simulink subsystem "MPC3_opti"  (R2023b)
settings: Solver=VariableStepAuto  StartTime=0.0  StopTime=10.0  RelTol=1e-3
undefined symbols (not defined in the file): param_MPC3, param_robot, param_traj_data, param_weight_init
settings Model: Creator=emu  LastModifiedBy=emu

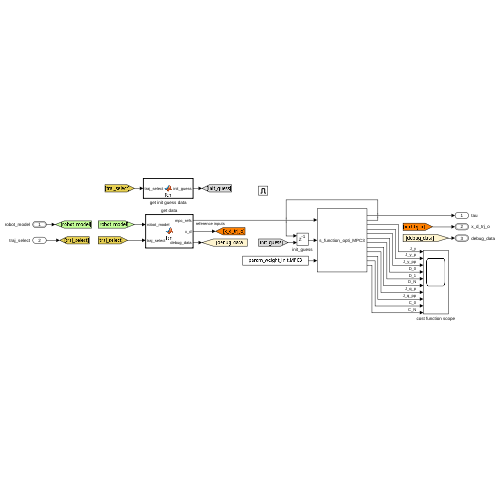
[thumbnail: Simulink's stored preview of the top-level diagram]
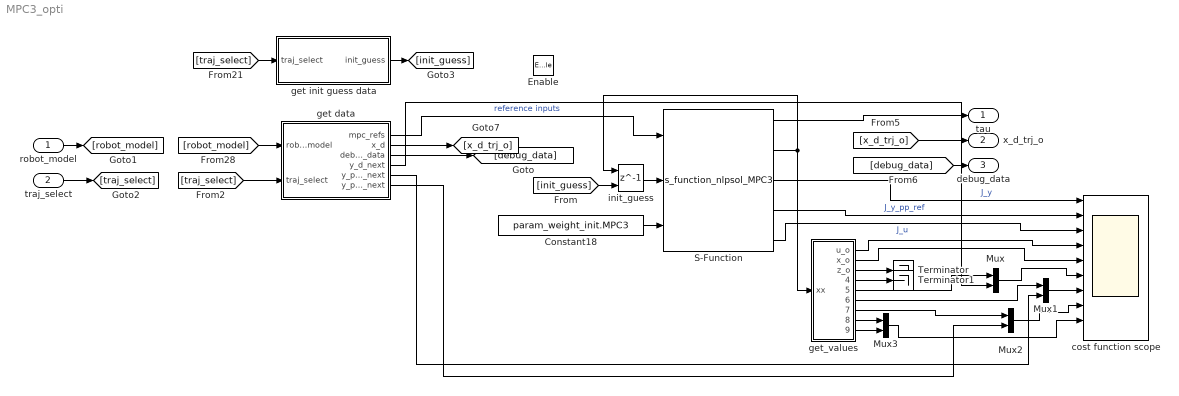
== system MPC3_opti ==
  robot_model : Inport  OutDataTypeStr=Bus: robot_model
  traj_select : Inport  Port=2
  Enable : EnablePort
  Constant18 : Constant  Value=param_weight_init.MPC3  VectorParams1D=off
  Mux{,1..3} (4 alike) : Mux  Inputs=2
  S-Function : S-Function  FunctionName=s_function_nlpsol_MPC3  Parameters='s_functions/MPC3.casadi', 'MPC3'  SFunctionModules='MPC3'  SFunctionDeploymentMode=off  EnableBusSupport=off
  Terminator : Terminator
  Terminator1 : Terminator
  cost function scope : Scope  NumInputPorts=10
  get data : MATLAB Function  TreatAsAtomicUnit=on
  get init guess data : MATLAB Function  TreatAsAtomicUnit=on
  get_values : MATLAB Function  TreatAsAtomicUnit=on
  init_guess : Delay  DelayLength=1  InitialConditionSource=Input port  InitialCondition=1
      settings: InputPortMap=u0,p4
  tau : Outport
  x_d_trj_o : Outport  Port=2  OutDataTypeStr=Bus: x_d
  debug_data : Outport  Port=3  OutDataTypeStr=Bus: debug_data_bus
  wires:
  get init guess data/1(init_guess) -> [init_guess]
  S-Function/2 -> init_guess/1, get_values/1(xx)
  [debug_data] -> debug_data/1
  get data/3(debug_data) -> [debug_data]
  get data/1(mpc_refs) -> S-Function/1  "reference inputs"
  S-Function/3 -> cost function scope/1  "J_y"
  [robot_model] -> get data/1(robot_model)
  S-Function/4 -> cost function scope/2  "J_y_pp_ref"
  [traj_select] -> get data/2(traj_select)
  [init_guess] -> init_guess/2
  Constant18/1 -> S-Function/3
  init_guess/1 -> S-Function/2
  [traj_select] -> get init guess data/1(traj_select)
  robot_model/1 -> [robot_model]
  [x_d_trj_o] -> x_d_trj_o/1
  get data/2(x_d) -> [x_d_trj_o]
  S-Function/1 -> tau/1
  traj_select/1 -> [traj_select]
  get_values/1(u_o) -> cost function scope/4
  get_values/2(x_o) -> cost function scope/5
  get_values/6(y_p_ref_next) -> Mux1/1
  get_values/7(y_pp_ref_next) -> Mux2/1
  get data/4(y_d_next) -> Mux/2
  get data/5(y_p_d_next) -> Mux1/2
  get data/6(y_pp_d_next) -> Mux2/2
  get_values/5(y_ref_next) -> Mux/1
  Mux1/1 -> cost function scope/7
  Mux2/1 -> cost function scope/8
  get_values/3(z_o) -> Terminator/1
  get_values/4(alpha_o) -> Terminator1/1
  Mux3/1 -> cost function scope/9
  get_values/8(y_N) -> Mux3/1
  get_values/9(y_ref_N) -> Mux3/2
  S-Function/5 -> cost function scope/3  "J_u"
  Mux/1 -> cost function scope/6

== matlab function MPC3_opti/get data ==
  settings: updateMethod=DISCRETE  sampleTime=param_global.Ta
  data: mpc_refs output; robot_model input Bus: robot_model; param_MPC3 parameter; x_d output Bus: x_d; debug_data output Bus: debug_data_bus; param_traj_data parameter; traj_select input; y_d_next output; y_p_d_next output; y_pp_d_next output
function [mpc_refs, x_d, debug_data, y_d_next, y_p_d_next, y_pp_d_next] = fcn(robot_model, param_MPC3, param_traj_data, traj_select)
persistent cnt;

if(isempty(cnt))
    cnt = 1;
end

param_MPC = param_MPC3;
N         = param_MPC.N;
N_step    = param_MPC.N_step;

% Parameters
q    = robot_model.q;      % generalized coordinates
q_p  = robot_model.q_p;  % time derivative of generalized coordinates
q_pp = robot_model.q_pp;
H    = robot_model.H;
J    = robot_model.J;
J_p  = robot_model.J_p;

% Current Pose of Endeffector
p = H(1:2,4);
p_p = J(1:2,1:2)*q_p;
p_pp = J(1:2,1:2)*q_pp + J_p(1:2,1:2)*q_p;

R = H(1:3,1:3);

% desired Orientation as Rotationmatrix
q_e = rotation2quaternion(R);

% Error of Position (translation) and first time derivative
q_err = quat_mult(q_e, quat_inv(param_traj_data.q_d(1:4, cnt, traj_select)));

x_k = [q;q_p];

% Assemble vector of recieved output measurements
p_d_traj    = param_traj_data.p_d(   1:3, cnt : N_step : cnt + (N)*N_step, traj_select);
p_d_p_traj  = param_traj_data.p_d_p( 1:3, cnt : N_step : cnt + (N)*N_step, traj_select);
p_d_pp_traj = param_traj_data.p_d_pp(1:3, cnt : N_step : cnt + (N)*N_step, traj_select);

y_ref    = p_d_traj(   1:2, 1 + (0:N) ); %       y1,   y2,   ... yN
y_ref_p  = p_d_p_traj( 1:2, 1 + (0:N) ); %       y1p,  y2p,  ... yNp
y_ref_pp = p_d_pp_traj(1:2, 1 + (0:N) ); % y0pp, y1pp, y2pp, ... yN-1pp

z_0 = [y_ref(:,1); y_ref_p(:,1)];
%z_0 = [p; p_p]; % aktuelle Position ist problematisch und führt zu instab.

y_d_next = y_ref(:,2);
y_p_d_next = y_ref_p(:, 2);
y_pp_d_next = y_ref_pp(:, 2);

cnt = cnt+1;

%% Reference out

mpc_refs = [x_k(:); z_0(:); y_ref(:); y_ref_p(:); y_ref_pp(:)]';

%% TRAJECTORY OUT
x_d.p_d       = p_d_traj(1:3,1);    %y0
x_d.p_d_p     = p_d_p_traj(1:3,1);  %y0p
x_d.p_d_pp    = p_d_pp_traj(1:3,1); %y0pp
x_d.q_d       = [0; 0; 0; 0];
x_d.omega_d   = [0; 0; 0];
x_d.omega_d_p = [0; 0; 0];

%% DEBUG
debug_data.p    = p(1:2);
debug_data.p_p  = p_p(1:2);
debug_data.p_pp = p_pp(1:2);
debug_data.rot_x_err = q_err(2);
debug_data.rot_y_err = q_err(3);
debug_data.rot_z_err = q_err(4);

== matlab function MPC3_opti/get init guess data ==
  data: traj_select input; param_MPC3_init_guess parameter; init_guess output
function init_guess  = fcn(traj_select, param_MPC3_init_guess)

init_guess = param_MPC3_init_guess.init_guess(traj_select, :);

== matlab function MPC3_opti/get_values ==
  data: xx input; u_o output; x_o output; z_o output; alpha_o output; param_MPC3 parameter; param_robot parameter; y_ref_next output; y_p_ref_next output; y_pp_ref_next output; y_N output; y_ref_N output
function [u_o, x_o, z_o, alpha_o, y_ref_next, y_p_ref_next, y_pp_ref_next, y_N, y_ref_N] = fcn(xx, param_MPC3, param_robot)

n = param_robot.n_DOF;

len_u     = n*  (param_MPC3.N  );
len_x     = 2*n*(param_MPC3.N+1);
len_z     = 2*n*(param_MPC3.N+1);
len_alpha = n*  (param_MPC3.N+1);


u = xx(1:len_u);

offset = len_u;

x = xx(offset + (1:len_x));

offset = len_u + len_x;

z = xx(offset + (1:len_z));

offset = len_u + len_x + len_z;

alpha = xx(offset + (1:len_alpha));

u_o = u(1:2);
x_o = x(1:4);
z_o = z(1:4);
alpha_o = alpha(1:2);

y_ref_next = z(4+(1:2));
y_p_ref_next = z(4+(3:4));
y_pp_ref_next = alpha(2+(1:2));

q_N = x(end-3:end-2);
H_N = hom_transform_endeffector(q_N, param_robot);

y_N = H_N(1:2, 4)';
y_ref_N = z(end-3:end-2);
